simulink model "temperature_control_withoutPID"  (R2016b)
settings: Solver=VariableStepAuto  StartTime=0.0  StopTime=10.0  RelTol=1e-3
libraries: fl_lib x3, nesl_utility x3
settings Model: Creator=sphoorthy nadimpalli  LastModifiedBy=sphoorthy nadimpalli

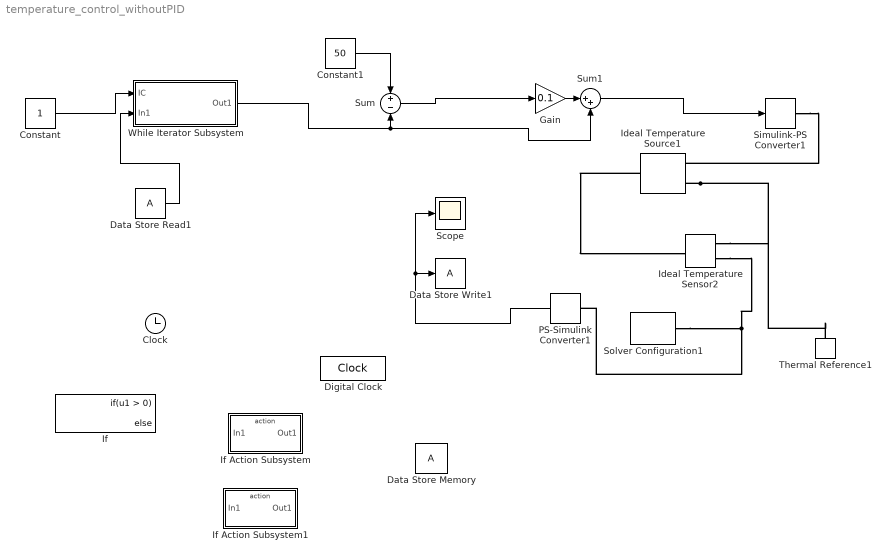
== system temperature_control_withoutPID ==
  Clock : Clock
  Constant : Constant
  Constant1 : Constant  Value=50
  Data Store Memory : DataStoreMemory  ReadBeforeWriteMsg=warning  WriteAfterWriteMsg=warning  WriteAfterReadMsg=warning  ShowAdditionalParam=off
  Data Store Read1 : DataStoreRead
  Data Store Write1 : DataStoreWrite
  Digital Clock : DigitalClock
  Gain : Gain  Gain=0.1
  Ideal Temperature Sensor2 : fl_lib/Thermal/Thermal Sensors/Ideal Temperature Sensor
  Ideal Temperature Source1 : fl_lib/Thermal/Thermal Sources/Ideal Temperature Source
  If : If
  If Action Subsystem : Subsystem  TreatAsAtomicUnit=on
  If Action Subsystem1 : Subsystem  TreatAsAtomicUnit=on
  PS-Simulink Converter1 : nesl_utility/PS-Simulink Converter  PhysicalDomain=network_engine_domain  SubClassName=ps_output  LeftPortType=input  RightPortType=output  PseudoPeriodic=off  Frequencies=[]  Unit=1  AffineConversion=off
  Scope : Scope
  Simulink-PS Converter1 : nesl_utility/Simulink-PS Converter  PhysicalDomain=network_engine_domain  SubClassName=ps_input  LeftPortType=input  RightPortType=output  PseudoPeriodic=off  Frequencies=[]  NoiseDistribution=none  NoiseParameters=[]  Unit=1  AffineConversion=off  InputFiltering=off  SimscapeFilterOrder=1  InputFilterTimeConstant=0.001  UdotUserProvided=1
  Solver Configuration1 : nesl_utility/Solver Configuration  PhysicalDomain=network_engine_domain  SubClassName=solver  LeftPortType=input  RightPortType=generic  Accelerate=off  Tones=[]  Harmonics=[]  SimulateNoise=off  Profile=off  UseLocalSampling=off  EnableSwitchedLinearOptims=on  FrequencyDomain=off  UseCCode=off  RelTol=0.001  AbsTol=1e-06  MinStep=1e-09  ToWorkspace=off  RevertToSquareIcSolve=off  NumHomotopyIterations=100  PhasorMode=off  PhasorModeNumHarmonics=1  OverrideAbsTol=off  DoDC=off  ResidualTolerance=1e-09  UseLocalSolver=off  LocalSolverChoice=NE_BACKWARD_EULER_ADVANCER  LocalSolverSampleTime=0.001  DoFixedCost=off  MaxNonlinIter=3  MaxModeIter=2  LinearAlgebra=Sparse  DelaysMemoryBudget=1024  AutomaticFiltering=on  FilteringTimeConstant=0.001
  Sum : Sum  Inputs=+-
  Sum1 : Sum  Inputs=|++
  Thermal Reference1 : fl_lib/Thermal/Thermal Elements/Thermal Reference
  While Iterator Subsystem : Subsystem  TreatAsAtomicUnit=on
  wires:
  Constant/1 -> While Iterator Subsystem/1(IC)
  Constant1/1 -> Sum/1
  PS-Simulink Converter1/1 -> Scope/1, Data Store Write1/1
  Sum/1 -> Gain/1
  Gain/1 -> Sum1/1
  Sum1/1 -> Simulink-PS Converter1/1
  Data Store Read1/1 -> While Iterator Subsystem/2(In1)
  While Iterator Subsystem/1(Out1) -> Sum1/2, Sum/2
  connections:
  Ideal Temperature Source1/RConn2 -- Thermal Reference1/LConn1 -- Ideal Temperature Sensor2/RConn1
  Ideal Temperature Sensor2/RConn2 -- PS-Simulink Converter1/LConn1 -- Solver Configuration1/RConn1
  Ideal Temperature Source1/LConn1 -- Ideal Temperature Sensor2/LConn1
  Simulink-PS Converter1/RConn1 -- Ideal Temperature Source1/RConn1

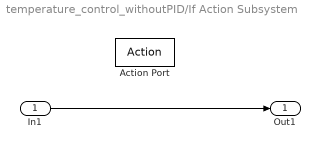
== system temperature_control_withoutPID/If Action Subsystem ==
  In1 : Inport
  Action Port : ActionPort
  Out1 : Outport
  wires:
  In1/1 -> Out1/1

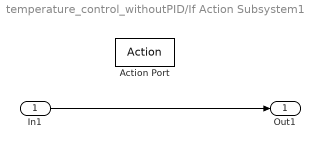
== system temperature_control_withoutPID/If Action Subsystem1 ==
  In1 : Inport
  Action Port : ActionPort
  Out1 : Outport
  wires:
  In1/1 -> Out1/1

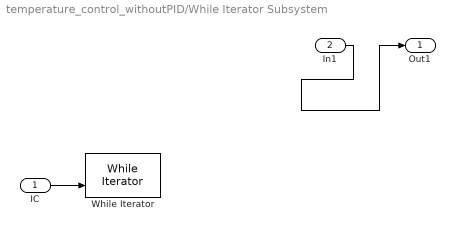
== system temperature_control_withoutPID/While Iterator Subsystem ==
  IC : Inport
  In1 : Inport  Port=2
  While Iterator : WhileIterator
  Out1 : Outport
  wires:
  IC/1 -> While Iterator/2
  ? -> While Iterator/1
  In1/1 -> Out1/1
